simulink model "test_var"  (R2023b)
settings: Solver=FixedStepAuto  StartTime=0.0  StopTime=1e-5  FixedStep=1e-7  RelTol=1e-3  EnableMultiTasking=on
values from neighbouring files (symbols this model uses):
  idx_rand = randi([1, num_C*num_R], 1, 1)    [code_lsandtrain.m]
  in = data.in    [code_lsandtrain.m]
  out = data.out    [code_lsandtrain.m]
settings Model: Creator=Jhchen  LastModifiedBy=Jhchen
settings DataIOCC: ReturnWorkspaceOutputs=off
settings OptimizationCC: DefaultParameterBehavior=Inlined  UseDivisionForNetSlopeComputation=on  GainParamInheritBuiltInType=on  UseFloatMulNetSlope=on  DefaultUnderspecifiedDataType=single  InlineInvariantSignals=on  PassReuseOutputArgsThreshold=0  ZeroExternalMemoryAtStartup=off  ZeroInternalMemoryAtStartup=off  EfficientFloat2IntCast=on  LifeSpan=1  MaxStackSize=64  OptimizeBlockOrder=speed  DifferentSizesBufferReuse=on
settings DebuggingCC: ParameterTunabilityLossMsg=error
settings HardwareCC: ProdLongLongMode=on
settings ModelReferenceCC: ModelReferenceNumInstancesAllowed=Single
settings SFSimCC: MATLABDynamicMemAlloc=off
settings RTWCC: GenerateReport=on  Toolchain=Texas Instruments Code Composer Studio (C2000)  LaunchReport=on  TargetLang=C++
settings CodeAppCC: ForceParamTrailComments=on  OperatorAnnotations=on
settings GRTTargetCC: TargetLangStandard=C++11 (ISO)  CombineSignalStateStructs=on  MatFileLogging=off  CodeInterfacePackaging=C++ class  SupportVariableSizeSignals=on

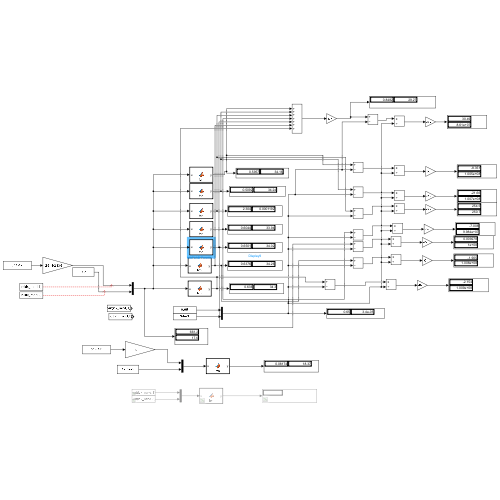
[thumbnail: Simulink's stored preview of the top-level diagram]
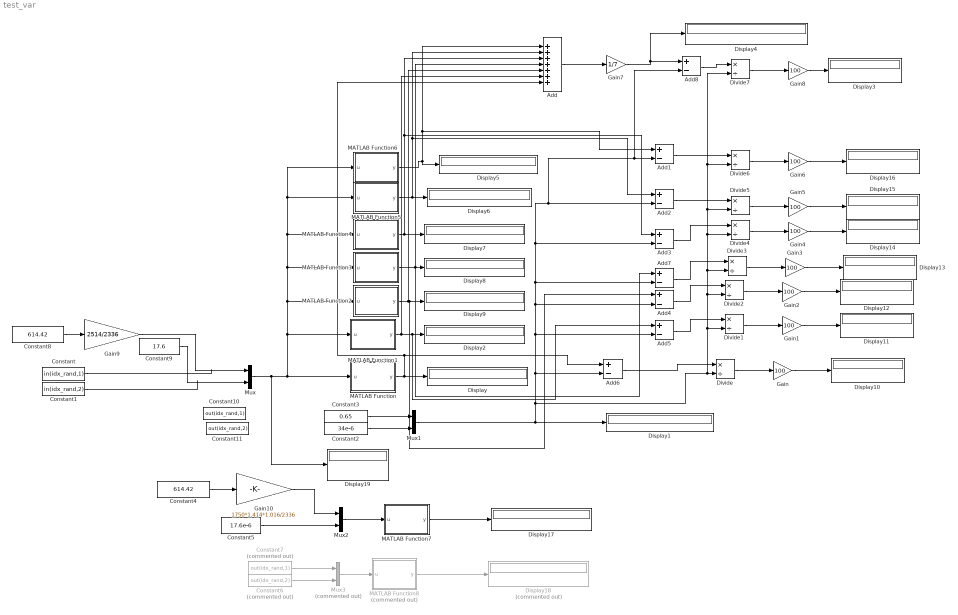
== system test_var ==
  Add : Sum  Inputs=7
  Add{1..8} (8 alike) : Sum  Inputs=+-
  Constant : Constant  Value=in(idx_rand,1)
  Constant1 : Constant  Value=in(idx_rand,2)
  Constant10 : Constant  Value=out(idx_rand,1)
  Constant11 : Constant  Value=out(idx_rand,2)
  Constant2 : Constant  Value=34e-6
  Constant3 : Constant  Value=0.65
  Constant4 : Constant  Value=614.42
  Constant5 : Constant  Value=17.6e-6
  Constant6 : Constant  Commented=on  Value=out(idx_rand,2)
  Constant7 : Constant  Commented=on  Value=out(idx_rand,1)
  Constant8 : Constant  Value=614.42
  Constant9 : Constant  Value=17.6
  Display{,1..17,19} (19 alike) : Display
  Display18 : Display  Commented=on
  Divide{,1..7} (8 alike) : Product  Inputs=*/
  Gain{,1..6,8} (8 alike) : Gain  Gain=100
  Gain10 : Gain  Gain=1750*1.414*1.016/2336
  Gain7 : Gain  Gain=1/7
  Gain9 : Gain  Gain=2514/2336
  MATLAB Function : MATLAB Function  TreatAsAtomicUnit=on
  MATLAB Function1 : MATLAB Function  TreatAsAtomicUnit=on
  MATLAB Function2 : MATLAB Function  TreatAsAtomicUnit=on
  MATLAB Function3 : MATLAB Function  TreatAsAtomicUnit=on
  MATLAB Function4 : MATLAB Function  TreatAsAtomicUnit=on
  MATLAB Function5 : MATLAB Function  TreatAsAtomicUnit=on
  MATLAB Function6 : MATLAB Function  TreatAsAtomicUnit=on
  MATLAB Function7 : MATLAB Function  TreatAsAtomicUnit=on
  MATLAB Function8 : MATLAB Function  Commented=on  TreatAsAtomicUnit=on
  Mux : Mux  Inputs=2
  Mux1 : Mux  Inputs=2
  Mux2 : Mux  Inputs=2
  Mux3 : Mux  Commented=on  Inputs=2
  wires:
  Constant8/1 -> Gain9/1
  MATLAB Function/1(y) -> Add/7, Add6/1, Display/1
  Constant3/1 -> Mux1/1
  Constant2/1 -> Mux1/2
  Mux1/1 -> Divide7/2, Divide6/2, Divide5/2, Divide4/2, Divide3/2, Divide2/2, Divide1/2, Divide/2, Add8/2, Add1/2, Add2/2, Add3/2, Add7/2, Add4/2, Add5/2, Add6/2, Display1/1
  MATLAB Function1/1(y) -> Add5/1, Display2/1, Add/6
  Mux/1 -> Display19/1, MATLAB Function6/1(u), MATLAB Function5/1(u), MATLAB Function4/1(u), MATLAB Function3/1(u), MATLAB Function2/1(u), MATLAB Function1/1(u), MATLAB Function/1(u)
  MATLAB Function2/1(y) -> Add/5, Add4/1, Display9/1
  MATLAB Function3/1(y) -> Add/4, Display8/1, Add7/1
  MATLAB Function4/1(y) -> Add/3, Add3/1, Display7/1
  MATLAB Function5/1(y) -> Add/2, Add2/1, Display6/1
  MATLAB Function6/1(y) -> Add/1, Add1/1, Display5/1
  Add6/1 -> Divide/1
  Divide/1 -> Gain/1
  Gain/1 -> Display10/1
  Gain1/1 -> Display11/1
  Divide1/1 -> Gain1/1
  Divide2/1 -> Gain2/1
  Gain2/1 -> Display12/1
  Gain3/1 -> Display13/1
  Divide3/1 -> Gain3/1
  Divide4/1 -> Gain4/1
  Gain4/1 -> Display14/1
  Gain5/1 -> Display15/1
  Divide5/1 -> Gain5/1
  Divide6/1 -> Gain6/1
  Gain6/1 -> Display16/1
  Add1/1 -> Divide6/1
  Add2/1 -> Divide5/1
  Add3/1 -> Divide4/1
  Add7/1 -> Divide3/1
  Add4/1 -> Divide2/1
  Add5/1 -> Divide1/1
  Add/1 -> Gain7/1
  Gain7/1 -> Add8/1, Display4/1
  Divide7/1 -> Gain8/1
  Gain8/1 -> Display3/1
  Add8/1 -> Divide7/1
  Constant5/1 -> Mux2/2
  Constant4/1 -> Gain10/1
  MATLAB Function7/1(y) -> Display17/1
  Mux2/1 -> MATLAB Function7/1(u)
  Constant6/1 -> Mux3/2
  Constant7/1 -> Mux3/1
  Mux3/1 -> MATLAB Function8/1(u)
  MATLAB Function8/1(y) -> Display18/1
  Constant/1 -> ?
  Constant1/1 -> ?
  Gain10/1 -> Mux2/1
  Gain9/1 -> Mux/1
  Constant9/1 -> Mux/2

== matlab function test_var/MATLAB Function ==
  data: u input; y output
function y = fcn(u)

y = predict16(u);

== matlab function test_var/MATLAB Function2 ==
  data: u input; y output
function y = fcn(u)

y = predict2(u);

== matlab function test_var/MATLAB Function3 ==
  data: u input; y output
function y = fcn(u)

y = predict3(u);

== matlab function test_var/MATLAB Function4 ==
  data: u input; y output
function y = fcn(u)

y = predict4(u);

== matlab function test_var/MATLAB Function5 ==
  data: u input; y output
function y = fcn(u)

y = predict5(u);

== matlab function test_var/MATLAB Function6 ==
  data: u input; y output
function y = fcn(u)

y = predict6(u);

== matlab function test_var/MATLAB Function7 ==
  data: u input; y output
function y = fcn(u)

y = predict16(u);

== matlab function test_var/MATLAB Function8 ==
  data: u input; y output
function y = fcn(u)

y = predict1(u);

== matlab function test_var/MATLAB Function1 ==
  data: u input; y output
function y = fcn(u)

y = predict1(u);
